simulink model "modelSquare"  (Simulink 10.0)
settings: Solver=ode23tb  StartTime=0.0  StopTime=1000.0  MaxStep=1  RelTol=1e-3  EnableMultiTasking=on
libraries: LemmingToolbox x6
settings Model: Creator=langmo  LastModifiedBy=unknown
settings DataIOCC: LimitDataPoints=on  SignalLoggingSaveFormat=ModelDataLogs
settings OptimizationCC: ExpressionDepthLimit=2147483647  InitFltsAndDblsToZero=on
settings DebuggingCC: SolverPrmCheckMsg=warning  FcnCallInpInsideContextMsg=warning  StateNameClashWarn=warning
settings SFSimCC: SimUseLocalCustomCode=on  CustomCodeUndefinedFunction=FilterOut
settings RTWCC: RTWUseLocalCustomCode=on

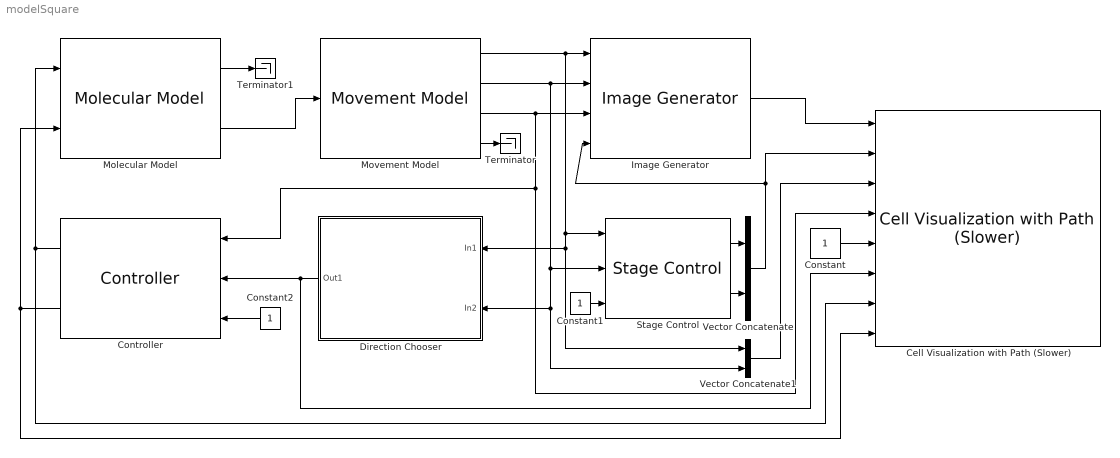
== system modelSquare ==
  Cell Visualization with Path (Slower) : LemmingToolbox/Cell Visualization with Path (Slower)  SystemSampleTime=-1  outputFilename=outWithPath.avi  imageDim=[1344,1024]  binning=2  maxNumCells=1  coneWidth=150  coneAngle=pi/4  pathLength=30  frameWidth=131  frameHeight=100  maxPathDimensions=[-4, -4, 14, 14]  referenceX=[0, 0, 10, 10, 0]  referenceY=[0, 10, 10, 0, 0]  sampleTimes=[0.3, 0.1]
  Constant : Constant  OutDataTypeStr=uint32
  Constant1 : Constant
  Constant2 : Constant  OutDataTypeStr=boolean
  Controller : LemmingToolbox/Controller  sampleTimes=[0.3, 0.1]  controller=@controllerHysteresis
  Direction Chooser : Subsystem
      mask Display:
      | text(0.3,0.1,'Direction Chooser');
      | color('blue');
      | port_label('input', 1, 'X-Pos');
      | port_label('input', 2, 'Y-Pos');
      | port_label('output', 1, 'phi_sh');
  Image Generator : LemmingToolbox/Image Generator  binning=2  numCells=1  sampleTime=[0.3, 0.1]
  Molecular Model : LemmingToolbox/Molecular Model  molecModel=Spiro  controlledCheSpecies=CheY  cheSpeciesAttachedTo=CheX-PhyB & PIF3-Anker  asp=1e-3  useOrgParameters=off  CheX=42  AnkerProt=57  Anker=80
  Movement Model : LemmingToolbox/Movement Model  imageDim=[1344,1024]  binning=2  pixelSize=6.45 / 40  initialCondition=[0, 0, pi/3]  sampleTimes=[0.03, 0]
  Stage Control : LemmingToolbox/Stage Control  SystemSampleTime=-1  activate=on  controlMicroscope=off  cooldown=0  border=0.25  initialCondition=[-0.5, -0.5]  sampleTimes=[0.3, 0.1]
  Terminator : Terminator
  Terminator1 : Terminator
  Vector Concatenate : Concatenate  ConcatenateDimension=2
  Vector Concatenate1 : Concatenate  Mode=Multidimensional array  ConcatenateDimension=2
  wires:
  Stage Control/2 -> Vector Concatenate/2
  Stage Control/1 -> Vector Concatenate/1
  Molecular Model/2 -> Movement Model/1
  Movement Model/1 -> Image Generator/1, Stage Control/1, Vector Concatenate1/1, Direction Chooser/1(In1)
  Movement Model/2 -> Image Generator/2, Stage Control/2, Vector Concatenate1/2, Direction Chooser/2(In2)
  Movement Model/3 -> Image Generator/3, Controller/1, Cell Visualization with Path (Slower)/4
  Vector Concatenate/1 -> Image Generator/4, Cell Visualization with Path (Slower)/2
  Image Generator/1 -> Cell Visualization with Path (Slower)/1
  Vector Concatenate1/1 -> Cell Visualization with Path (Slower)/3
  Constant/1 -> Cell Visualization with Path (Slower)/5
  Movement Model/4 -> Terminator/1
  Molecular Model/1 -> Terminator1/1
  Constant1/1 -> Stage Control/3
  Constant2/1 -> Controller/3
  Direction Chooser/1(Out1) -> Controller/2, Cell Visualization with Path (Slower)/6
  Controller/1 -> Molecular Model/1, Cell Visualization with Path (Slower)/7
  Controller/2 -> Molecular Model/2, Cell Visualization with Path (Slower)/8

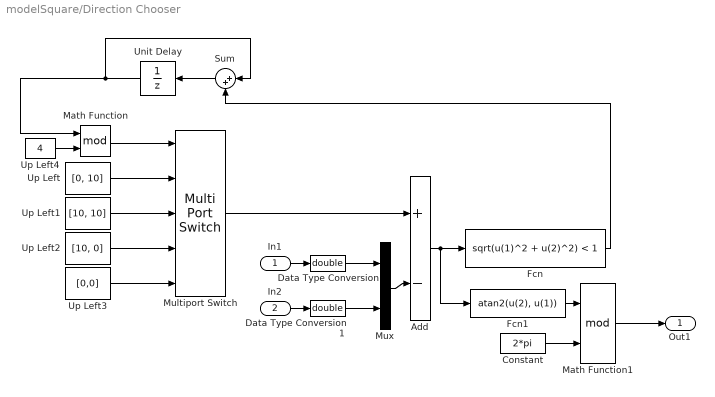
== system modelSquare/Direction Chooser ==
  In1 : Inport
  In2 : Inport  Port=2
  Add : Sum  Inputs=+-
  Constant : Constant  Value=2*pi
  Data Type Conversion : DataTypeConversion  OutDataTypeStr=double  SampleTime=0.3
  Data Type Conversion1 : DataTypeConversion  OutDataTypeStr=double  SampleTime=0.3
  Fcn : Fcn  Expr=sqrt(u(1)^2 + u(2)^2) < 1
  Fcn1 : Fcn  Expr=atan2(u(2), u(1))
  Math Function : Math  Operator=mod  SaturateOnIntegerOverflow=on
  Math Function1 : Math  Operator=mod  SaturateOnIntegerOverflow=on
  Multiport Switch : MultiPortSwitch  DataPortOrder=Zero-based contiguous  Inputs=4  zeroidx=on
  Mux : Mux  Inputs=2
  Sum : Sum  Inputs=|++
  Unit Delay : UnitDelay  SampleTime=0.3
  Up Left : Constant  Value=[0, 10]
  Up Left1 : Constant  Value=[10, 10]
  Up Left2 : Constant  Value=[10, 0]
  Up Left3 : Constant  Value=[0,0]
  Up Left4 : Constant  Value=4
  Out1 : Outport
  wires:
  Up Left/1 -> Multiport Switch/2
  Up Left3/1 -> Multiport Switch/5
  Up Left2/1 -> Multiport Switch/4
  Up Left1/1 -> Multiport Switch/3
  In2/1 -> Data Type Conversion1/1
  In1/1 -> Data Type Conversion/1
  Sum/1 -> Unit Delay/1
  Unit Delay/1 -> Sum/1, Math Function/1
  Up Left4/1 -> Math Function/2
  Math Function/1 -> Multiport Switch/1
  Multiport Switch/1 -> Add/1
  Mux/1 -> Add/2
  Add/1 -> Fcn/1, Fcn1/1
  Fcn/1 -> Sum/2
  Data Type Conversion/1 -> Mux/1
  Data Type Conversion1/1 -> Mux/2
  Fcn1/1 -> Math Function1/1
  Constant/1 -> Math Function1/2
  Math Function1/1 -> Out1/1
